simulink model "PID_centerlineTracking"  (R2023b)
settings: Solver=VariableStepAuto  StartTime=0.0  StopTime=Te  RelTol=1e-3
values from neighbouring files (symbols this model uses):
  Ts = 0.1    [ScriptBoot.m]    (also in ScriptBoot_TEST.m)
undefined symbols (not defined in the file or in its folder): accMAX, brakeMAX, driving, egoCarID, jerkMAX, lr, m, position0, turnAngleMAX, turnAngleRateMAX, velocity0
libraries: drivingscenarioandsensors x7, robotcorelib x2, autolibshared x1, sensorinslib x1
(part 3 of 3)

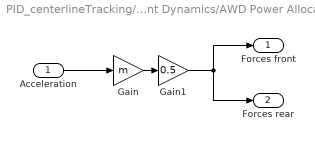
== system PID_centerlineTracking/Agent Dynamics/AWD Power Allocation ==
  Acceleration : Inport
  Gain : Gain  Gain=m
  Gain1 : Gain  Gain=0.5
  Forces front : Outport  VectorParamsAs1DForOutWhenUnconnected=off
  Forces rear : Outport  Port=2  VectorParamsAs1DForOutWhenUnconnected=off
  wires:
  Gain/1 -> Gain1/1
  Gain1/1 -> Forces front/1, Forces rear/1
  Acceleration/1 -> Gain/1

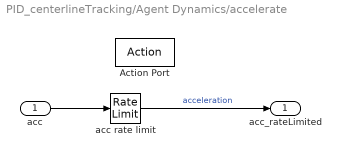
== system PID_centerlineTracking/Agent Dynamics/accelerate ==
  acc : Inport
  Action Port : ActionPort  ActionPortLabel=if(u1 > 0)
  acc rate limit : RateLimiter  RisingSlewLimit=jerkMAX  FallingSlewLimit=-jerkMAX  SampleTimeMode=inherited
  acc_rateLimited : Outport
  wires:
  acc/1 -> acc rate limit/1
  acc rate limit/1 -> acc_rateLimited/1  "acceleration"

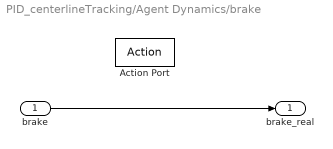
== system PID_centerlineTracking/Agent Dynamics/brake ==
  brake : Inport
  Action Port : ActionPort  ActionPortLabel=else
  brake_real : Outport
  wires:
  brake/1 -> brake_real/1

== matlab function PID_centerlineTracking/Environment/Pack Ego Actor ==
  data: pos input; a output Bus: BusActors1Actors size=1; vel input; yaw input; yawRate input; ActorID input
function a = packEgo(pos,vel,yaw,yawRate,ActorID)
% Pack ego information into a single ego actor bus
%
% Imoprtant note:
% Output is a bus of type BusActorsActors. This is the same bus used by the
% Scenario Reader to output an individual actor. If you change the
% output bus name of Scenario Reader change the output bus name here
% as well by clicking on 'Edit Data' in the menu above.

a = struct(...
    'ActorID',ActorID,...
    'Position', [pos(1) pos(2) 0], ...
    'Velocity', [vel(1) vel(2) 0], ...
    'Roll', 0, ...
    'Pitch', 0, ...
    'Yaw', yaw, ...
    'AngularVelocity', [0 0 yawRate]);
